simulink model "Furuta_Control_Fixed_Arm"  (R2017a)
settings: Solver=FixedStepAuto  StartTime=0.0  StopTime=30  FixedStep=Ts  RelTol=1e-3
PreLoadFcn:
  | %myBusDef
StartFcn:
  | % Full path to the block
  | %blk = 'Furuta_Control/Bus Creator';
  | 
  | % Attach the event listener
  | %h = add_exec_event_listener(blk, ...
  | %         'PostOutputs', @displayBusdata);
values from neighbouring files (symbols this model uses):
  omega_n = 8.4908    [Furuta_Constants.m]
  zeta = 0.0145    [Furuta_Constants.m]
settings Model: Creator=Marcelo  LastModifiedBy=Felipe
settings SolverCC: ZeroCrossControl=DisableAll
settings DebuggingCC: ParameterOverflowMsg=warning  BusObjectLabelMismatch=error
settings ModelReferenceCC: ModelReferenceMinAlgLoopOccurrences=on
settings ConfigComp: PLC_TargetIDE=codesys23  PLC_GenerateReport=off

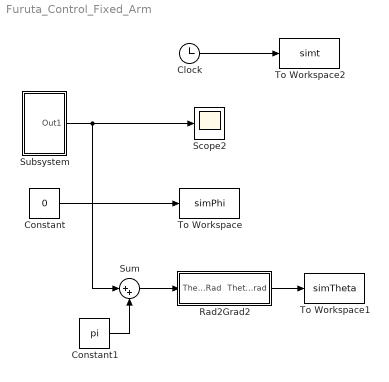
== system Furuta_Control_Fixed_Arm ==
  Clock : Clock
  Constant : Constant  Value=0
  Constant1 : Constant  Value=pi
  Rad2Grad2 : Subsystem
  Scope2 : Scope
  Subsystem : Subsystem
  Sum : Sum  Inputs=|++
  To Workspace : ToWorkspace  VariableName=simPhi  SampleTime=-1
      settings: Save2DSignal=2-D array (concatenate along first dimension)
  To Workspace1 : ToWorkspace  VariableName=simTheta  SampleTime=-1
      settings: Save2DSignal=2-D array (concatenate along first dimension)
  To Workspace2 : ToWorkspace  VariableName=simt  SampleTime=-1
      settings: Save2DSignal=2-D array (concatenate along first dimension)
  wires:
  Rad2Grad2/1(ThetaGrad) -> To Workspace1/1
  Clock/1 -> To Workspace2/1
  Constant/1 -> To Workspace/1
  Sum/1 -> Rad2Grad2/1(ThetaRad)
  Constant1/1 -> Sum/2
  Subsystem/1(Out1) -> Scope2/1, Sum/1

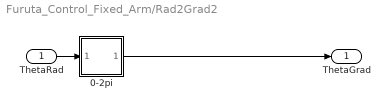
== system Furuta_Control_Fixed_Arm/Rad2Grad2 ==
  ThetaRad : Inport
  0-2pi : Subsystem
  ThetaGrad : Outport
  wires:
  ThetaRad/1 -> 0-2pi/1(In1)
  0-2pi/1(Out1) -> ThetaGrad/1

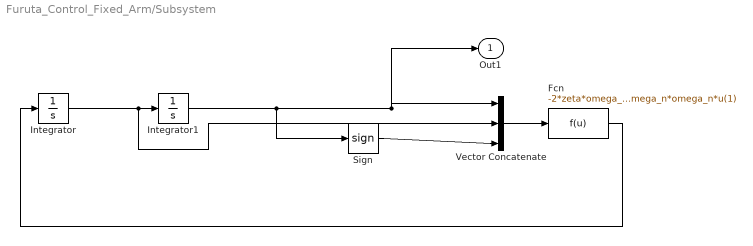
== system Furuta_Control_Fixed_Arm/Subsystem ==
  Fcn : Fcn  Expr=-2*zeta*omega_n*u(2)-omega_n*omega_n*u(1)
  Integrator : Integrator
  Integrator1 : Integrator  InitialCondition=15*pi/180
  Sign : Signum
  Vector Concatenate : Concatenate  NumInputs=3
  Out1 : Outport
  wires:
  Integrator/1 -> Vector Concatenate/2, Integrator1/1
  Vector Concatenate/1 -> Fcn/1
  Integrator1/1 -> Out1/1, Vector Concatenate/1, Sign/1
  Fcn/1 -> Integrator/1
  Sign/1 -> Vector Concatenate/3

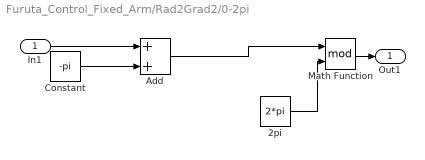
== system Furuta_Control_Fixed_Arm/Rad2Grad2/0-2pi ==
  In1 : Inport
  2pi : Constant  Value=2*pi
  Add : Sum
  Constant : Constant  Value=-pi
  Math Function : Math  Operator=mod  SaturateOnIntegerOverflow=on
  Out1 : Outport
  wires:
  Math Function/1 -> Out1/1
  2pi/1 -> Math Function/2
  Constant/1 -> Add/2
  In1/1 -> Add/1
  Add/1 -> Math Function/1
